simulink model "DUs_Exp"  (R2022b)
settings: Solver=ode4  StartTime=0.0  StopTime=0.3  RelTol=1e-3
model workspace (MAT data in the model file):
  C = 0.0011
  E = 75
  L = 0.001
  R = 10000000
libraries: simulink x30, spsSeriesRLCBranchLib x6, spsCurrentMeasurementLib x4, spsVoltageMeasurementLib x4, spsControlledVoltageSourceLib x2, spsDiodeLib x2, spsMosfetLib x2, spsPWMGeneratorDCDCLib x2, spsStairGeneratorLib x2, spsControlledCurrentSourceLib x1, rllib x1, spspowerguiLib x1
settings Model: Creator=86177  LastModifiedBy=Sweet_J

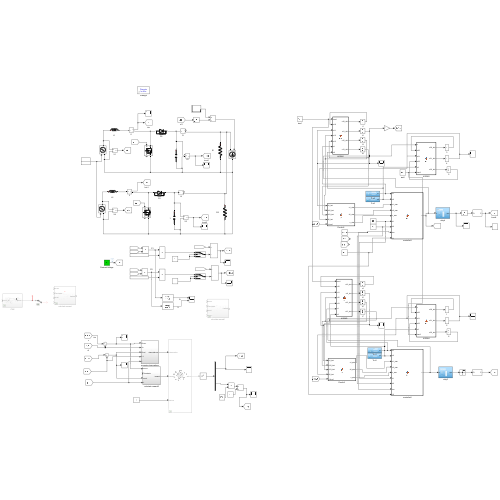
[thumbnail: Simulink's stored preview of the top-level diagram]
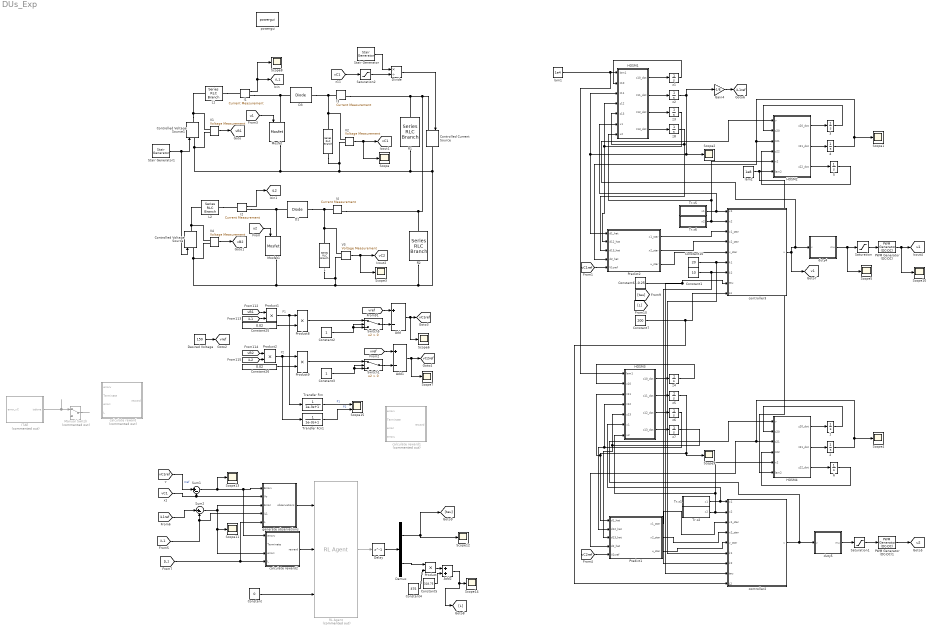
== system DUs_Exp ==
  note: P2
  note: P1
  " " : spsSeriesRLCBranchLib/Series RLC Branch  LConnTagsString=__new0  RConnTagsString=__new0  BranchType=C  Resistance=0.1  Inductance=1e-3  SetiL0=off  InitialCurrent=0  Capacitance=C  Setx0=on  InitialVoltage=150  Measurements=None
  " 1" : spsSeriesRLCBranchLib/Series RLC Branch  LConnTagsString=__new0  RConnTagsString=__new0  BranchType=C  Resistance=0.1  Inductance=1e-3  SetiL0=off  InitialCurrent=0  Capacitance=C  Setx0=off  InitialVoltage=150  Measurements=None
  {1..6} (6 alike) : Integrator  InitialCondition=-5
  Add : Sum  Inputs=+-
  Add1 : Sum  Inputs=+-
  Add2 : Sum
  Constant : Constant  Value=0
  Constant1 : Constant  Value=10
  Constant10 : Constant  Value=20
  Constant2 : Constant
  Constant25 : Constant  Value=0.02
  Constant26 : Constant  Value=0.02
  Constant3 : Constant
  Constant4 : Constant  Value=375
  Constant5 : Constant  Value=318.75
  Constant6 : Constant  Value=-0.25
  Constant7 : Constant  Value=200
  Controlled Current Source : spsControlledCurrentSourceLib/Controlled Current Source  Initialize=on  Source_Type=AC  Amplitude=0  Phase=0  Frequency=0  Measurements=None
  Controlled Voltage Source : spsControlledVoltageSourceLib/Controlled Voltage Source  Initialize=on  Source_Type=DC  Amplitude=0  Phase=0  Frequency=0  Measurements=None
  Controlled Voltage Source1 : spsControlledVoltageSourceLib/Controlled Voltage Source  Initialize=on  Source_Type=DC  Amplitude=0  Phase=0  Frequency=0  Measurements=None
  D1 : spsDiodeLib/Diode  Ron=0.00001  Lon=0  Vf=0  IC=0  UseSnubber=off  Rs=500000  Cs=10e-9  Measurements=off
  D3 : spsDiodeLib/Diode  Ron=0.00001  Lon=0  Vf=0  IC=0  UseSnubber=off  Rs=500000  Cs=10e-9  Measurements=off
  Delay : Delay  DelayLength=1
  Demux : Demux  Outputs=2
  Desired Voltage : Constant  Value=150
  Divide : Product  Inputs=*/
  Gain4 : Gain  Gain=-1/E
  HOSM1 : MATLAB Function  TreatAsAtomicUnit=on
  HOSM2 : MATLAB Function  TreatAsAtomicUnit=on
  HOSM3 : MATLAB Function  TreatAsAtomicUnit=on
  HOSM4 : MATLAB Function  TreatAsAtomicUnit=on
  I{1..4} (4 alike) : spsCurrentMeasurementLib/Current Measurement  PhasorSimulation=off  OutputType=Complex  PSBequivalent=0
  ITAE : Subsystem  Commented=on
  L1 : spsSeriesRLCBranchLib/Series RLC Branch  LConnTagsString=__new0  RConnTagsString=__new0  BranchType=L  Resistance=0.002  Inductance=L  SetiL0=off  InitialCurrent=0  Capacitance=1e-6  Setx0=off  InitialVoltage=0  Measurements=None
  L2 : spsSeriesRLCBranchLib/Series RLC Branch  LConnTagsString=__new0  RConnTagsString=__new0  BranchType=L  Resistance=0.002  Inductance=L  SetiL0=off  InitialCurrent=0  Capacitance=1e-6  Setx0=off  InitialVoltage=0  Measurements=None
  Manual Switch : ManualSwitch  Commented=on
  Mosfet : spsMosfetLib/Mosfet  Ron=0.01  Lon=0  Rd=0.01  Vfd=0  IC=0  Rs=1e5  Cs=inf  Measurements=on
  Mosfet1 : spsMosfetLib/Mosfet  Ron=0.01  Lon=0  Rd=0.01  Vfd=0  IC=0  Rs=1e5  Cs=inf  Measurements=on
  PWM Generator (DC-DC) : spsPWMGeneratorDCDCLib/PWM Generator (DC-DC)  Fsw=20000  Ts=1e-6
  PWM Generator (DC-DC)1 : spsPWMGeneratorDCDCLib/PWM Generator (DC-DC)  Fsw=20000  Ts=1e-6
  Predict1 : MATLAB Function  TreatAsAtomicUnit=on
  Predict2 : MATLAB Function  TreatAsAtomicUnit=on
  Product{,1..2,8..9} (5 alike) : Product
  R1 : spsSeriesRLCBranchLib/Series RLC Branch  LConnTagsString=__new0  RConnTagsString=__new0  BranchType=R  Resistance=R  Inductance=5e-3  SetiL0=off  InitialCurrent=0  Capacitance=1e-6  Setx0=off  InitialVoltage=0  Measurements=None
  R2 : spsSeriesRLCBranchLib/Series RLC Branch  LConnTagsString=__new0  RConnTagsString=__new0  BranchType=R  Resistance=R  Inductance=5e-3  SetiL0=off  InitialCurrent=0  Capacitance=1e-6  Setx0=off  InitialVoltage=0  Measurements=None
  RL Agent : rllib/RL Agent  Commented=on  Agent=agent  ExternalActionAsInput=off  ProvideLastAction=off  ProvideCumRwd=off  TreatAsDirectFeedthrough=on  UseStrictObservationDataTypes=off
  Saturation : Saturate  UpperLimit=0.99  LowerLimit=0.01
  Saturation1 : Saturate  UpperLimit=0.99  LowerLimit=0.01
  Saturation2 : Saturate  UpperLimit=700  LowerLimit=1
  Scope{,1..14} (15 alike) : Scope
  Scope15 : Scope  NumInputPorts=2
  Stair Generator : spsStairGeneratorLib/Stair Generator  t=[0, 0.11, 0.23]  e=[800,100,400]  Ts=0
  Stair Generator1 : spsStairGeneratorLib/Stair Generator  t=[0,0.2,0.25]  e=[75,75,75]  Ts=0
  Sum1 : Sum  Inputs=|+-
  Sum2 : Sum  Inputs=|+-
  Switch1 : Switch  Criteria=u2 > Threshold  SaturateOnIntegerOverflow=off  InputSameDT=off
  Switch5 : Switch  Criteria=u2 > Threshold  SaturateOnIntegerOverflow=off  InputSameDT=off
  Tr.x1 : Subsystem
  Tr.x2 : Subsystem
  Tr.x5 : Subsystem
  Tr.x6 : Subsystem
  Transfer Fcn : TransferFcn  Denominator=[1e-3 1]
  Transfer Fcn1 : TransferFcn  Denominator=[1e-3 1]
  V{1..4} (4 alike) : spsVoltageMeasurementLib/Voltage Measurement  PhasorSimulation=off  OutputType=Complex  PSBequivalent=0
  calculate reward : Subsystem  Commented=on
  calculate reward1 : Subsystem  Commented=on
  calculate reward2 : Subsystem
  controller2 : MATLAB Function  TreatAsAtomicUnit=on
  controller3 : MATLAB Function  TreatAsAtomicUnit=on
  duty4 : Subsystem
  duty5 : Subsystem
  generate observations : Subsystem
  lam1 : Constant  Value=1e4
  lam2 : Constant  Value=1e8
  powergui : spspowerguiLib/powergui  Priority=1  SimulationMode=Discrete  SampleTime=1e-6  frequency=60  Iterations=50  frequencyindice=0  Pbase=100e6  ErrMax=1e-4  UnitsV=kV  UnitsW=MW  buscounter=0  FunctionMessages=off  echomessages=off  EnableUseOfTLC=off  CurrentSourceSwitches=off  DisableSnubberDevices=off  DisableRonSwitches=off  DisableVfSwitches=off  DisplayEquations=off  AutomaticDiscreteSolvers=off  SolverType=Tustin/Backward Euler (TBE)  Interpol=off  ExternalGateDelay=off  methode=off  Ts=100  x0status=blocks  SPID=on  SwTol=0  HookPort=off  NonlinearTolerance=1e-4  nMaxIteration=100  ContinueOnMaxIteration=off  RestoreLinks=warning  ResistiveCurrentMeasurement=off  Frange=[0:2:500]  Ylog=off  Xlog=on  ShowGrid=off  save=off  variable=ZData  structure=0  ZoomFFT=off  StartTime=0.0  cycles=1  DisplayStyle=1  fundamental=60  FreqAxis=off  MaxFrequency=1000  frequencyindicesteady=1  RmsSteady=1  display=off
  z1 : Integrator  InitialCondition=-1
  z2 : Integrator  InitialCondition=-200
  z{3,6..8} (4 alike) : Integrator
  z4 : Integrator  InitialCondition=-1
  z5 : Integrator  InitialCondition=-200
  tag scope: iL1=global, iL1ref=global, iL2=global, u1=global, u2=global, v1=global, vB1=global, vB2=global, vC1=global, vC1ref=global, vC2=global, vC2ref=global, vref=global
  wires:
  Manual Switch/1 -> ?
  Add2/1 -> [L], Scope14/1
  RL Agent/1 -> Delay/1
  Sum1/1 -> Scope13/1, calculate reward2/1(errorv), generate observations/1(Errorv)
  ITAE/1(isdone) -> Manual Switch/1
  4/1 -> Scope1/1, Predict2/4(d2_hat), HOSM2/3(z21)
  I1/1 -> [iL1], Scope8/1
  V2/1 -> [vC1], Scope/1
  Stair Generator1/1 -> Controlled Voltage Source/1, Controlled Voltage Source1/1
  Divide/1 -> Controlled Current Source/1
  Gain4/1 -> [iL1ref]
  [vC1ref] -> Sum1/1  "Vref"
  calculate reward2/1(reward) -> RL Agent/2
  Tr.x1/1(x1) -> HOSM3/6(x1), controller2/1(x1)
  generate observations/1(observations) -> RL Agent/1
  [vC1] -> Sum1/2, generate observations/2(Vo)
  Constant3/1 -> Switch1/3, Switch1/2
  [iL1] -> generate observations/4(iL1), Sum2/2
  Sum2/1 -> calculate reward2/3(errori), Scope11/1, generate observations/3(Errori)
  [vC1] -> Saturation2/1
  duty5/1(mu) -> Saturation1/1
  Saturation/1 -> PWM Generator (DC-DC)/1
  Add1/1 -> [vC2ref], Scope7/1
  Predict2/3(u_star) -> controller3/5(v_star)
  HOSM3/1(z10_dot) -> z4/1
  HOSM2/2(z21_dot) -> 4/1
  Constant10/1 -> controller2/6(k1), controller3/6(k1)
  controller3/1(v) -> duty4/1(v), HOSM2/1(v), [v1]
  Saturation1/1 -> PWM Generator (DC-DC)1/1
  Add/1 -> [vC1ref], Scope6/1
  Saturation2/1 -> Divide/2
  duty4/1(mu) -> Scope5/1, Saturation/1
  Constant25/1 -> Product8/2
  Tr.x6/1(x2) -> HOSM1/7(x2), HOSM2/5(x2), controller3/2(x2)
  Predict1/3(u_star) -> controller2/5(v_star)
  z4/1 -> HOSM3/2(z10)
  [vC2ref] -> Predict1/5(V2cref)
  V1/1 -> [vB1]
  HOSM1/4(z13_dot) -> z8/1
  I2/1 -> [iL2]
  Predict2/2(x2_star) -> controller3/4(x2_star)
  Desired Voltage/1 -> [vref]
  3/1 -> HOSM2/2(z20)
  z3/1 -> Predict2/2(d12_hat), HOSM1/4(z12)
  HOSM2/3(z22_dot) -> 5/1
  HOSM2/1(z20_dot) -> 3/1
  5/1 -> HOSM2/4(z22)
  z1/1 -> HOSM1/2(z10)
  HOSM1/2(z11_dot) -> z2/1
  [iL1ref] -> Sum2/1
  PWM Generator (DC-DC)1/1 -> [u2]
  z8/1 -> Predict2/3(d13_hat), HOSM1/5(z13)
  Constant26/1 -> Product9/2
  Predict2/1(x1_star) -> controller3/3(x1_star)
  [vB1] -> Product1/1
  [vB2] -> Product2/1
  Constant2/1 -> Switch5/2, Switch5/3
  HOSM4/3(z22_dot) -> 6/1
  HOSM1/1(z10_dot) -> z1/1
  [iL1] -> Product1/2
  PWM Generator (DC-DC)/1 -> [u1], Scope10/1
  Switch5/1 -> Add/2
  [vref] -> Add1/1
  Product2/1 -> Product9/1, Transfer Fcn1/1
  Stair Generator/1 -> Divide/1
  6/1 -> HOSM4/4(z22)
  lam1/1 -> HOSM3/1(lam1), HOSM1/1(lam1)
  1/1 -> HOSM4/2(z20)
  z6/1 -> HOSM3/4(z12), Predict1/2(d12_hat)
  HOSM3/3(z12_dot) -> z6/1
  V4/1 -> [vB2]
  HOSM1/3(z12_dot) -> z3/1
  Switch1/1 -> Add1/2
  Product9/1 -> Switch1/1
  [iL2] -> Product2/2
  Product8/1 -> Switch5/1
  Predict1/2(x2_star) -> controller2/4(x2_star)
  Constant1/1 -> controller2/7(k2), controller3/7(k2)
  HOSM3/2(z11_dot) -> z5/1
  HOSM4/2(z21_dot) -> 2/1
  Tr.x5/1(x1) -> HOSM1/6(x1), controller3/1(x1)
  2/1 -> HOSM4/3(z21), Predict1/4(d2_hat), Scope4/1
  z7/1 -> HOSM3/5(z13), Predict1/3(d13_hat)
  V3/1 -> [vC2], Scope3/1
  controller2/1(v) -> HOSM4/1(v), duty5/1(v)
  Product1/1 -> Product8/1, Transfer Fcn/1
  Tr.x2/1(x2) -> controller2/2(x2), HOSM4/5(x2), HOSM3/7(x2)
  [vref] -> Add/1
  HOSM4/1(z20_dot) -> 1/1
  Predict1/1(x1_star) -> controller2/3(x1_star)
  [vC1ref] -> Predict2/5(V1cref)
  z2/1 -> Scope2/1, HOSM1/3(z11), Predict2/1(d1_hat), Gain4/1
  HOSM3/4(z13_dot) -> z7/1
  z5/1 -> Scope9/1, Predict1/1(d1_hat), HOSM3/3(z11)
  [u1] -> Mosfet/1
  lam2/1 -> HOSM4/6(lam2), HOSM2/6(lam2)
  Demux/1 -> Scope12/1, [tau]
  [u2] -> Mosfet1/1
  Delay/1 -> Demux/1
  Demux/2 -> Product/1
  Constant4/1 -> Product/2
  Product/1 -> Add2/1
  Constant5/1 -> Add2/2
  Constant6/1 -> controller3/8(tau), controller2/8(tau)
  Constant/1 -> RL Agent/3
  Transfer Fcn/1 -> Scope15/1  "P1"
  Transfer Fcn1/1 -> Scope15/2  "P2"
  [L] -> calculate reward2/4(L), generate observations/5(L)
  Constant7/1 -> controller2/9(L2), controller3/9(L1)
  connections:
  Controlled Voltage Source1/RConn1 -- V1/LConn1 -- L1/LConn1
  L2/LConn1 -- Controlled Voltage Source/RConn1 -- V4/LConn1
  V2/LConn1 -- D3/RConn1 -- I3/LConn1 -- " "/LConn1
  " 1"/LConn1 -- V3/LConn1 -- D1/RConn1 -- I4/LConn1
  I1/RConn1 -- D3/LConn1 -- Mosfet/LConn1
  Mosfet1/LConn1 -- I2/RConn1 -- D1/LConn1
  L2/RConn1 -- I2/LConn1
  L1/RConn1 -- I1/LConn1
  I3/RConn1 -- I4/RConn1 -- R2/LConn1 -- Controlled Current Source/LConn1 -- R1/LConn1
  R2/RConn1 -- R1/RConn1 -- Controlled Voltage Source1/LConn1 -- V1/LConn2 -- Mosfet/RConn1 -- " "/RConn1 -- V2/LConn2 -- Controlled Current Source/RConn1 -- V3/LConn2 -- " 1"/RConn1 -- Controlled Voltage Source/LConn1 -- V4/LConn2 -- Mosfet1/RConn1

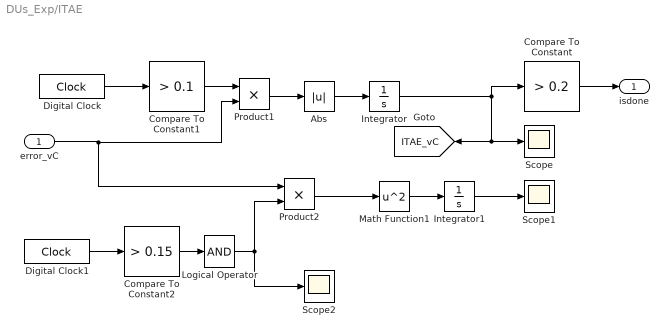
== system DUs_Exp/ITAE ==
  error_vC : Inport
  Abs : Abs  ZeroCross=off  SaturateOnIntegerOverflow=off
  Compare To Constant : simulink/Logic and Bit Operations/Compare To Constant  relop=>  const=0.2  OutDataTypeStr=boolean  ZeroCross=off
  Compare To Constant1 : simulink/Logic and Bit Operations/Compare To Constant  relop=>  const=0.1  OutDataTypeStr=boolean  ZeroCross=off
  Compare To Constant2 : simulink/Logic and Bit Operations/Compare To Constant  relop=>  const=0.15  OutDataTypeStr=boolean  ZeroCross=off
  Digital Clock : DigitalClock  SampleTime=1e-6
  Digital Clock1 : DigitalClock  SampleTime=1e-6
  Integrator : Integrator
  Integrator1 : Integrator
  Logical Operator : Logic  Inputs=1  AllPortsSameDT=off  OutDataTypeStr=boolean
  Math Function1 : Math  Operator=square
  Product1 : Product
  Product2 : Product
  Scope : Scope
  Scope1 : Scope
  Scope2 : Scope
  isdone : Outport
  tag scope: ITAE_vC=global
  wires:
  Abs/1 -> Integrator/1
  Digital Clock/1 -> Compare To Constant1/1
  Product1/1 -> Abs/1
  Compare To Constant/1 -> isdone/1
  Math Function1/1 -> Integrator1/1
  Integrator/1 -> Scope/1, [ITAE_vC], Compare To Constant/1
  Compare To Constant1/1 -> Product1/1
  Integrator1/1 -> Scope1/1
  Compare To Constant2/1 -> Logical Operator/1
  Digital Clock1/1 -> Compare To Constant2/1
  Logical Operator/1 -> Scope2/1, Product2/2
  error_vC/1 -> Product2/1, Product1/2
  Product2/1 -> Math Function1/1

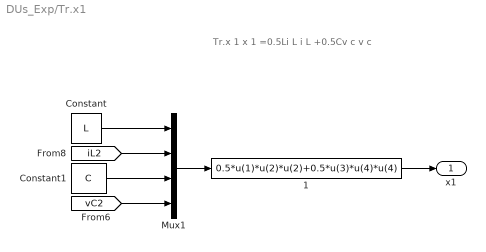
== system DUs_Exp/Tr.x1 ==
  note: Tr.x 1
      | x 1 =0.5Li L i L +0.5Cv c v c
  1 : Fcn  Expr=0.5*u(1)*u(2)*u(2)+0.5*u(3)*u(4)*u(4)
  Constant : Constant  Value=L
  Constant1 : Constant  Value=C
  Mux1 : Mux
  x1 : Outport  VectorParamsAs1DForOutWhenUnconnected=off
  wires:
  1/1 -> x1/1
  Mux1/1 -> 1/1
  Constant/1 -> Mux1/1
  [iL2] -> Mux1/2
  Constant1/1 -> Mux1/3
  [vC2] -> Mux1/4

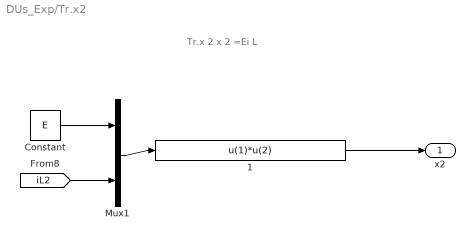
== system DUs_Exp/Tr.x2 ==
  note: Tr.x 2
      | x 2 =Ei L
  1 : Fcn  Expr=u(1)*u(2)
  Constant : Constant  Value=E
  Mux1 : Mux  Inputs=2
  x2 : Outport  VectorParamsAs1DForOutWhenUnconnected=off
  wires:
  [iL2] -> Mux1/2
  Mux1/1 -> 1/1
  1/1 -> x2/1
  Constant/1 -> Mux1/1

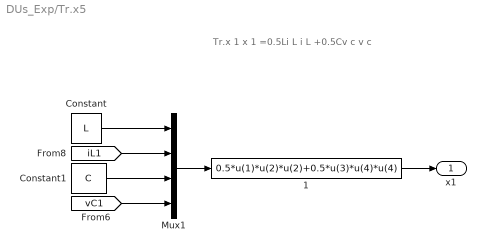
== system DUs_Exp/Tr.x5 ==
  note: Tr.x 1
      | x 1 =0.5Li L i L +0.5Cv c v c
  1 : Fcn  Expr=0.5*u(1)*u(2)*u(2)+0.5*u(3)*u(4)*u(4)
  Constant : Constant  Value=L
  Constant1 : Constant  Value=C
  Mux1 : Mux
  x1 : Outport  VectorParamsAs1DForOutWhenUnconnected=off
  wires:
  1/1 -> x1/1
  Mux1/1 -> 1/1
  Constant/1 -> Mux1/1
  [iL1] -> Mux1/2
  Constant1/1 -> Mux1/3
  [vC1] -> Mux1/4

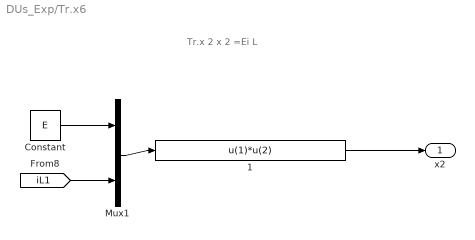
== system DUs_Exp/Tr.x6 ==
  note: Tr.x 2
      | x 2 =Ei L
  1 : Fcn  Expr=u(1)*u(2)
  Constant : Constant  Value=E
  Mux1 : Mux  Inputs=2
  x2 : Outport  VectorParamsAs1DForOutWhenUnconnected=off
  wires:
  [iL1] -> Mux1/2
  Mux1/1 -> 1/1
  1/1 -> x2/1
  Constant/1 -> Mux1/1

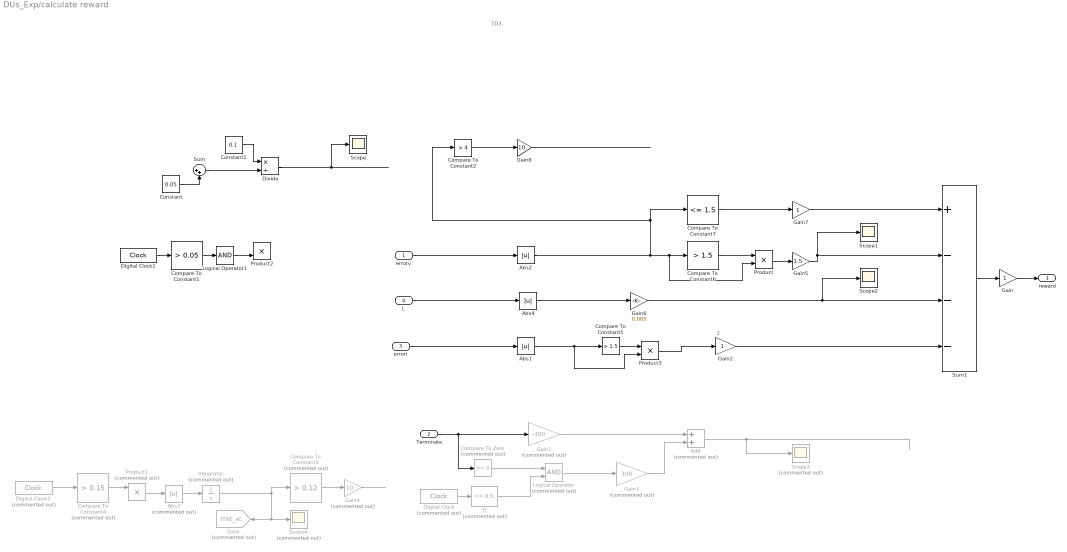
== system DUs_Exp/calculate reward ==
  note: 2
  note: TD3
  errorv : Inport
  Terminate : Inport  Port=2
  errori : Inport  Port=3
  L : Inport  Port=4
  Abs1 : Abs  ZeroCross=off  SaturateOnIntegerOverflow=off
  Abs2 : Abs  ZeroCross=off  SaturateOnIntegerOverflow=off
  Abs3 : Abs  Commented=on  ZeroCross=off  SaturateOnIntegerOverflow=off
  Abs4 : Abs  ZeroCross=off  SaturateOnIntegerOverflow=off
  Add : Sum  Commented=on
  Compare To Constant1 : simulink/Logic and Bit Operations/Compare To Constant  relop=>  const=0.05  OutDataTypeStr=boolean  ZeroCross=off
  Compare To Constant2 : simulink/Logic and Bit Operations/Compare To Constant  relop=>  const=4  OutDataTypeStr=boolean
  Compare To Constant3 : simulink/Logic and Bit Operations/Compare To Constant  Commented=on  relop=>  const=0.12  OutDataTypeStr=boolean  ZeroCross=off
  Compare To Constant4 : simulink/Logic and Bit Operations/Compare To Constant  Commented=on  relop=>  const=0.15  OutDataTypeStr=boolean  ZeroCross=off
  Compare To Constant5 : simulink/Logic and Bit Operations/Compare To Constant  relop=>  const=1.5  OutDataTypeStr=boolean
  Compare To Constant6 : simulink/Logic and Bit Operations/Compare To Constant  relop=>  const=1.5  OutDataTypeStr=boolean  ZeroCross=off
  Compare To Constant7 : simulink/Logic and Bit Operations/Compare To Constant  relop=<=  const=1.5  OutDataTypeStr=boolean  ZeroCross=off
  Compare To Zero : simulink/Logic and Bit Operations/Compare To Zero  Commented=on  relop===  OutDataTypeStr=boolean
  Constant : Constant  Value=0.05
  Constant1 : Constant  Value=0.1
  Digital Clock : DigitalClock  Commented=on  SampleTime=1e-6
  Digital Clock1 : DigitalClock  SampleTime=1e-6
  Digital Clock2 : DigitalClock  Commented=on  SampleTime=1e-6
  Divide : Product  Inputs=*/
  Gain : Gain
  Gain1 : Gain  Commented=on  Gain=-100
  Gain2 : Gain
  Gain3 : Gain  Commented=on  Gain=100
  Gain4 : Gain  Commented=on  Gain=10
  Gain5 : Gain  Gain=1.5
  Gain6 : Gain  Gain=0.005
  Gain7 : Gain
  Gain8 : Gain  Gain=10
  Goto : Goto  Commented=on  GotoTag=ITAE_vC  TagVisibility=global
  Integrator : Integrator  Commented=on
  Logical Operator : Logic  Commented=on  AllPortsSameDT=off  OutDataTypeStr=boolean
  Logical Operator1 : Logic  Inputs=1  AllPortsSameDT=off  OutDataTypeStr=boolean
  Product : Product
  Product1 : Product  Commented=on
  Product2 : Product
  Product3 : Product
  Scope : Scope
  Scope1 : Scope
  Scope2 : Scope
  Scope3 : Scope  Commented=on
  Scope4 : Scope  Commented=on
  Sum : Sum  Inputs=|++
  Sum1 : Sum  Inputs=+---  OutDataTypeStr=double
  Tf : simulink/Logic and Bit Operations/Compare To Constant  Commented=on  relop===  const=0.5  OutDataTypeStr=boolean  ZeroCross=off
  reward : Outport  VectorParamsAs1DForOutWhenUnconnected=off
  wires:
  Sum/1 -> Divide/2
  Constant/1 -> Sum/2
  Constant1/1 -> Divide/1
  Gain5/1 -> Sum1/2, Scope1/1
  Sum1/1 -> Gain/1
  Divide/1 -> Scope/1
  Gain/1 -> reward/1
  Gain1/1 -> Add/1
  Gain3/1 -> Add/2
  Compare To Zero/1 -> Logical Operator/1
  Digital Clock/1 -> Tf/1
  Terminate/1 -> Compare To Zero/1, Gain1/1
  Tf/1 -> Logical Operator/2
  Logical Operator/1 -> Gain3/1
  errori/1 -> Abs1/1
  Compare To Constant2/1 -> Gain8/1
  Gain2/1 -> Sum1/4
  Add/1 -> Scope3/1
  Logical Operator1/1 -> Product2/2
  Compare To Constant1/1 -> Logical Operator1/1
  Digital Clock1/1 -> Compare To Constant1/1
  errorv/1 -> Abs2/1
  Abs2/1 -> Compare To Constant2/1, Compare To Constant7/1, Product/2, Compare To Constant6/1
  Integrator/1 -> Goto/1, Scope4/1, Compare To Constant3/1
  Abs3/1 -> Integrator/1
  Digital Clock2/1 -> Compare To Constant4/1
  Compare To Constant3/1 -> Gain4/1
  Product1/1 -> Abs3/1
  Compare To Constant4/1 -> Product1/1
  Gain4/1 -> ?
  Gain8/1 -> ?
  Product3/1 -> Gain2/1
  L/1 -> Abs4/1
  Gain6/1 -> Sum1/3, Scope2/1
  Abs4/1 -> Gain6/1
  Abs1/1 -> Product3/2, Compare To Constant5/1
  Product/1 -> Gain5/1
  Compare To Constant7/1 -> Gain7/1
  Gain7/1 -> Sum1/1
  Compare To Constant6/1 -> Product/1
  Compare To Constant5/1 -> Product3/1

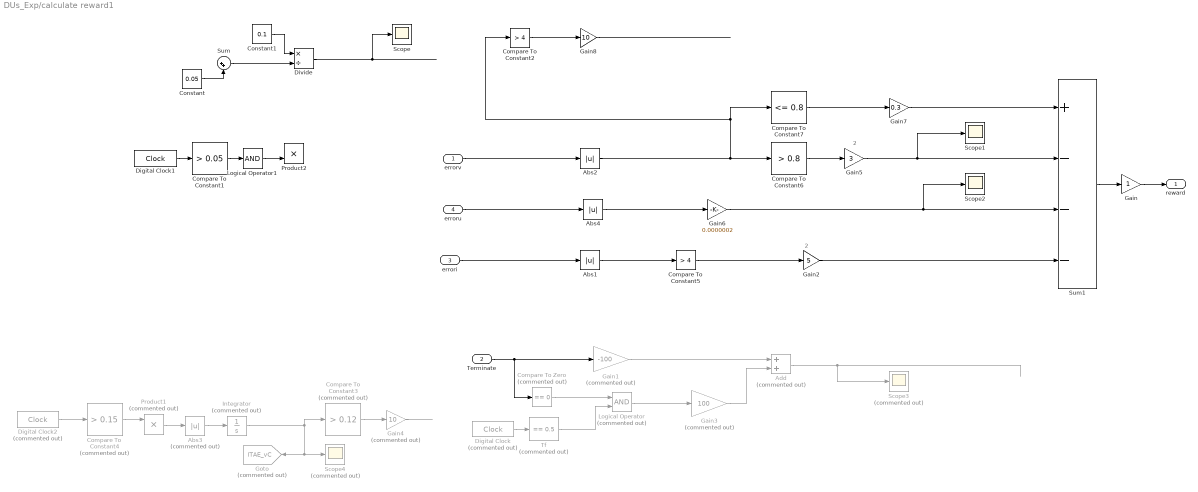
== system DUs_Exp/calculate reward1 ==
  note: 2
  note: 2
  errorv : Inport
  Terminate : Inport  Port=2
  errori : Inport  Port=3
  erroru : Inport  Port=4
  Abs1 : Abs  ZeroCross=off  SaturateOnIntegerOverflow=off
  Abs2 : Abs  ZeroCross=off  SaturateOnIntegerOverflow=off
  Abs3 : Abs  Commented=on  ZeroCross=off  SaturateOnIntegerOverflow=off
  Abs4 : Abs  ZeroCross=off  SaturateOnIntegerOverflow=off
  Add : Sum  Commented=on
  Compare To Constant1 : simulink/Logic and Bit Operations/Compare To Constant  relop=>  const=0.05  OutDataTypeStr=boolean  ZeroCross=off
  Compare To Constant2 : simulink/Logic and Bit Operations/Compare To Constant  relop=>  const=4  OutDataTypeStr=boolean
  Compare To Constant3 : simulink/Logic and Bit Operations/Compare To Constant  Commented=on  relop=>  const=0.12  OutDataTypeStr=boolean  ZeroCross=off
  Compare To Constant4 : simulink/Logic and Bit Operations/Compare To Constant  Commented=on  relop=>  const=0.15  OutDataTypeStr=boolean  ZeroCross=off
  Compare To Constant5 : simulink/Logic and Bit Operations/Compare To Constant  relop=>  const=4  OutDataTypeStr=boolean
  Compare To Constant6 : simulink/Logic and Bit Operations/Compare To Constant  relop=>  const=0.8  OutDataTypeStr=boolean  ZeroCross=off
  Compare To Constant7 : simulink/Logic and Bit Operations/Compare To Constant  relop=<=  const=0.8  OutDataTypeStr=boolean  ZeroCross=off
  Compare To Zero : simulink/Logic and Bit Operations/Compare To Zero  Commented=on  relop===  OutDataTypeStr=boolean
  Constant : Constant  Value=0.05
  Constant1 : Constant  Value=0.1
  Digital Clock : DigitalClock  Commented=on  SampleTime=1e-6
  Digital Clock1 : DigitalClock  SampleTime=1e-6
  Digital Clock2 : DigitalClock  Commented=on  SampleTime=1e-6
  Divide : Product  Inputs=*/
  Gain : Gain
  Gain1 : Gain  Commented=on  Gain=-100
  Gain2 : Gain  Gain=5
  Gain3 : Gain  Commented=on  Gain=100
  Gain4 : Gain  Commented=on  Gain=10
  Gain5 : Gain  Gain=3
  Gain6 : Gain  Gain=0.0000002
  Gain7 : Gain  Gain=0.3
  Gain8 : Gain  Gain=10
  Goto : Goto  Commented=on  GotoTag=ITAE_vC  TagVisibility=global
  Integrator : Integrator  Commented=on
  Logical Operator : Logic  Commented=on  AllPortsSameDT=off  OutDataTypeStr=boolean
  Logical Operator1 : Logic  Inputs=1  AllPortsSameDT=off  OutDataTypeStr=boolean
  Product1 : Product  Commented=on
  Product2 : Product
  Scope : Scope
  Scope1 : Scope
  Scope2 : Scope
  Scope3 : Scope  Commented=on
  Scope4 : Scope  Commented=on
  Sum : Sum  Inputs=|++
  Sum1 : Sum  Inputs=+---  OutDataTypeStr=double
  Tf : simulink/Logic and Bit Operations/Compare To Constant  Commented=on  relop===  const=0.5  OutDataTypeStr=boolean  ZeroCross=off
  reward : Outport  VectorParamsAs1DForOutWhenUnconnected=off
  wires:
  Gain7/1 -> Sum1/1
  Compare To Constant7/1 -> Gain7/1
  Compare To Constant6/1 -> Gain5/1
  Abs1/1 -> Compare To Constant5/1
  Abs4/1 -> Gain6/1
  Gain6/1 -> Scope2/1, Sum1/3
  erroru/1 -> Abs4/1
  Compare To Constant5/1 -> Gain2/1
  Gain8/1 -> ?
  Gain4/1 -> ?
  Compare To Constant4/1 -> Product1/1
  Product1/1 -> Abs3/1
  Compare To Constant3/1 -> Gain4/1
  Digital Clock2/1 -> Compare To Constant4/1
  Abs3/1 -> Integrator/1
  Integrator/1 -> Compare To Constant3/1, Scope4/1, Goto/1
  Abs2/1 -> Compare To Constant6/1, Compare To Constant7/1, Compare To Constant2/1
  errorv/1 -> Abs2/1
  Digital Clock1/1 -> Compare To Constant1/1
  Compare To Constant1/1 -> Logical Operator1/1
  Logical Operator1/1 -> Product2/2
  Add/1 -> Scope3/1
  Gain2/1 -> Sum1/4
  Compare To Constant2/1 -> Gain8/1
  errori/1 -> Abs1/1
  Logical Operator/1 -> Gain3/1
  Tf/1 -> Logical Operator/2
  Terminate/1 -> Gain1/1, Compare To Zero/1
  Digital Clock/1 -> Tf/1
  Compare To Zero/1 -> Logical Operator/1
  Gain3/1 -> Add/2
  Gain1/1 -> Add/1
  Gain/1 -> reward/1
  Divide/1 -> Scope/1
  Sum1/1 -> Gain/1
  Gain5/1 -> Scope1/1, Sum1/2
  Constant1/1 -> Divide/1
  Constant/1 -> Sum/2
  Sum/1 -> Divide/2

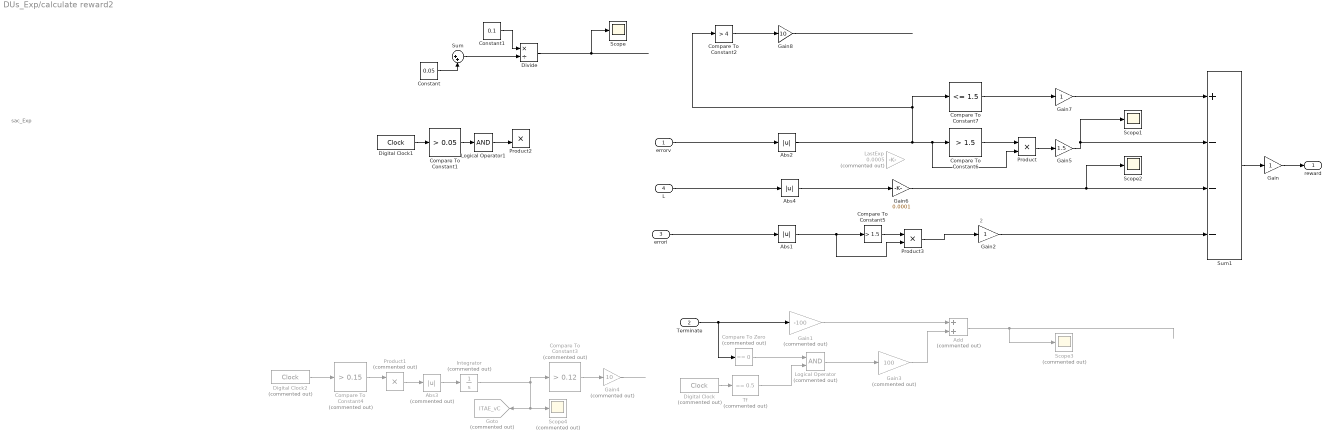
== system DUs_Exp/calculate reward2 ==
  note: sac_Exp
  note: 2
  errorv : Inport
  Terminate : Inport  Port=2
  errori : Inport  Port=3
  L : Inport  Port=4
  Abs1 : Abs  ZeroCross=off  SaturateOnIntegerOverflow=off
  Abs2 : Abs  ZeroCross=off  SaturateOnIntegerOverflow=off
  Abs3 : Abs  Commented=on  ZeroCross=off  SaturateOnIntegerOverflow=off
  Abs4 : Abs  ZeroCross=off  SaturateOnIntegerOverflow=off
  Add : Sum  Commented=on
  Compare To Constant1 : simulink/Logic and Bit Operations/Compare To Constant  relop=>  const=0.05  OutDataTypeStr=boolean  ZeroCross=off
  Compare To Constant2 : simulink/Logic and Bit Operations/Compare To Constant  relop=>  const=4  OutDataTypeStr=boolean
  Compare To Constant3 : simulink/Logic and Bit Operations/Compare To Constant  Commented=on  relop=>  const=0.12  OutDataTypeStr=boolean  ZeroCross=off
  Compare To Constant4 : simulink/Logic and Bit Operations/Compare To Constant  Commented=on  relop=>  const=0.15  OutDataTypeStr=boolean  ZeroCross=off
  Compare To Constant5 : simulink/Logic and Bit Operations/Compare To Constant  relop=>  const=1.5  OutDataTypeStr=boolean
  Compare To Constant6 : simulink/Logic and Bit Operations/Compare To Constant  relop=>  const=1.5  OutDataTypeStr=boolean  ZeroCross=off
  Compare To Constant7 : simulink/Logic and Bit Operations/Compare To Constant  relop=<=  const=1.5  OutDataTypeStr=boolean  ZeroCross=off
  Compare To Zero : simulink/Logic and Bit Operations/Compare To Zero  Commented=on  relop===  OutDataTypeStr=boolean
  Constant : Constant  Value=0.05
  Constant1 : Constant  Value=0.1
  Digital Clock : DigitalClock  Commented=on  SampleTime=1e-6
  Digital Clock1 : DigitalClock  SampleTime=1e-6
  Digital Clock2 : DigitalClock  Commented=on  SampleTime=1e-6
  Divide : Product  Inputs=*/
  Gain : Gain
  Gain1 : Gain  Commented=on  Gain=-100
  Gain2 : Gain
  Gain3 : Gain  Commented=on  Gain=100
  Gain4 : Gain  Commented=on  Gain=10
  Gain5 : Gain  Gain=1.5
  Gain6 : Gain  Gain=0.0001
  Gain7 : Gain
  Gain8 : Gain  Gain=10
  Goto : Goto  Commented=on  GotoTag=ITAE_vC  TagVisibility=global
  Integrator : Integrator  Commented=on
  LastExp : Gain  Commented=on  Gain=0.0005
  Logical Operator : Logic  Commented=on  AllPortsSameDT=off  OutDataTypeStr=boolean
  Logical Operator1 : Logic  Inputs=1  AllPortsSameDT=off  OutDataTypeStr=boolean
  Product : Product
  Product1 : Product  Commented=on
  Product2 : Product
  Product3 : Product
  Scope : Scope
  Scope1 : Scope
  Scope2 : Scope
  Scope3 : Scope  Commented=on
  Scope4 : Scope  Commented=on
  Sum : Sum  Inputs=|++
  Sum1 : Sum  Inputs=+---  OutDataTypeStr=double
  Tf : simulink/Logic and Bit Operations/Compare To Constant  Commented=on  relop===  const=0.5  OutDataTypeStr=boolean  ZeroCross=off
  reward : Outport  VectorParamsAs1DForOutWhenUnconnected=off
  wires:
  Compare To Constant5/1 -> Product3/1
  Compare To Constant6/1 -> Product/1
  Gain7/1 -> Sum1/1
  Compare To Constant7/1 -> Gain7/1
  Product/1 -> Gain5/1
  Abs1/1 -> Compare To Constant5/1, Product3/2
  Abs4/1 -> Gain6/1
  Gain6/1 -> Scope2/1, Sum1/3
  L/1 -> Abs4/1
  Product3/1 -> Gain2/1
  Gain8/1 -> ?
  Gain4/1 -> ?
  Compare To Constant4/1 -> Product1/1
  Product1/1 -> Abs3/1
  Compare To Constant3/1 -> Gain4/1
  Digital Clock2/1 -> Compare To Constant4/1
  Abs3/1 -> Integrator/1
  Integrator/1 -> Compare To Constant3/1, Scope4/1, Goto/1
  Abs2/1 -> Compare To Constant6/1, Product/2, Compare To Constant7/1, Compare To Constant2/1
  errorv/1 -> Abs2/1
  Digital Clock1/1 -> Compare To Constant1/1
  Compare To Constant1/1 -> Logical Operator1/1
  Logical Operator1/1 -> Product2/2
  Add/1 -> Scope3/1
  Gain2/1 -> Sum1/4
  Compare To Constant2/1 -> Gain8/1
  errori/1 -> Abs1/1
  Logical Operator/1 -> Gain3/1
  Tf/1 -> Logical Operator/2
  Terminate/1 -> Gain1/1, Compare To Zero/1
  Digital Clock/1 -> Tf/1
  Compare To Zero/1 -> Logical Operator/1
  Gain3/1 -> Add/2
  Gain1/1 -> Add/1
  Gain/1 -> reward/1
  Divide/1 -> Scope/1
  Sum1/1 -> Gain/1
  Gain5/1 -> Scope1/1, Sum1/2
  Constant1/1 -> Divide/1
  Constant/1 -> Sum/2
  Sum/1 -> Divide/2

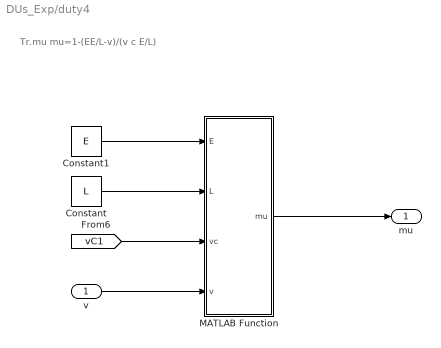
== system DUs_Exp/duty4 ==
  note: Tr.mu
      | mu=1-(EE/L-v)/(v c E/L)
  v : Inport
  Constant : Constant  Value=L
  Constant1 : Constant  Value=E
  MATLAB Function : MATLAB Function  TreatAsAtomicUnit=on
  mu : Outport  VectorParamsAs1DForOutWhenUnconnected=off
  wires:
  MATLAB Function/1(mu) -> mu/1
  v/1 -> MATLAB Function/4(v)
  [vC1] -> MATLAB Function/3(vc)
  Constant/1 -> MATLAB Function/2(L)
  Constant1/1 -> MATLAB Function/1(E)

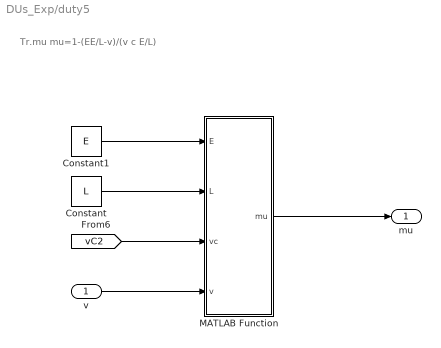
== system DUs_Exp/duty5 ==
  note: Tr.mu
      | mu=1-(EE/L-v)/(v c E/L)
  v : Inport
  Constant : Constant  Value=L
  Constant1 : Constant  Value=E
  MATLAB Function : MATLAB Function  TreatAsAtomicUnit=on
  mu : Outport  VectorParamsAs1DForOutWhenUnconnected=off
  wires:
  Constant1/1 -> MATLAB Function/1(E)
  Constant/1 -> MATLAB Function/2(L)
  [vC2] -> MATLAB Function/3(vc)
  v/1 -> MATLAB Function/4(v)
  MATLAB Function/1(mu) -> mu/1

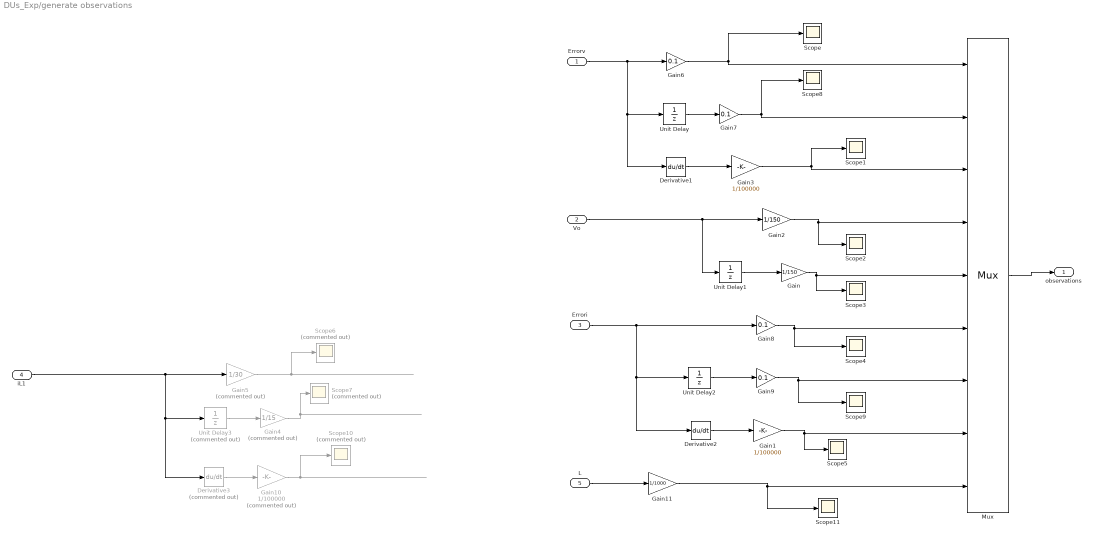
== system DUs_Exp/generate observations ==
  Errorv : Inport
  Vo : Inport  Port=2
  Errori : Inport  Port=3
  iL1 : Inport  Port=4
  L : Inport  Port=5
  Derivative1 : Derivative
  Derivative2 : Derivative
  Derivative3 : Derivative  Commented=on
  Gain : Gain  Gain=1/150
  Gain1 : Gain  Gain=1/100000
  Gain10 : Gain  Commented=on  Gain=1/100000
  Gain11 : Gain  Gain=1/1000
  Gain2 : Gain  Gain=1/150
  Gain3 : Gain  Gain=1/100000
  Gain4 : Gain  Commented=on  Gain=1/15
  Gain5 : Gain  Commented=on  Gain=1/30
  Gain{6..9} (4 alike) : Gain  Gain=0.1
  Mux : Mux  Inputs=9
  Scope{,1..5,8..9,11} (9 alike) : Scope
  Scope10 : Scope  Commented=on
  Scope6 : Scope  Commented=on
  Scope7 : Scope  Commented=on
  Unit Delay : UnitDelay  SampleTime=-1  HasFrameUpgradeWarning=on
  Unit Delay1 : UnitDelay  SampleTime=-1  HasFrameUpgradeWarning=on
  Unit Delay2 : UnitDelay  SampleTime=-1  HasFrameUpgradeWarning=on
  Unit Delay3 : UnitDelay  Commented=on  SampleTime=-1  HasFrameUpgradeWarning=on
  observations : Outport  VectorParamsAs1DForOutWhenUnconnected=off
  wires:
  Mux/1 -> observations/1
  Errorv/1 -> Derivative1/1, Unit Delay/1, Gain6/1
  Vo/1 -> Unit Delay1/1, Gain2/1
  Unit Delay1/1 -> Gain/1
  Gain/1 -> Scope3/1, Mux/5
  Derivative1/1 -> Gain3/1
  Gain3/1 -> Scope1/1, Mux/3
  Gain2/1 -> Scope2/1, Mux/4
  Gain1/1 -> Scope5/1, Mux/8
  Derivative2/1 -> Gain1/1
  Errori/1 -> Derivative2/1, Unit Delay2/1, Gain8/1
  Gain5/1 -> Scope6/1
  Gain4/1 -> Scope7/1
  Unit Delay3/1 -> Gain4/1
  Gain6/1 -> Scope/1, Mux/1
  Unit Delay/1 -> Gain7/1
  Gain7/1 -> Scope8/1, Mux/2
  Gain8/1 -> Scope4/1, Mux/6
  Unit Delay2/1 -> Gain9/1
  Gain9/1 -> Scope9/1, Mux/7
  Gain10/1 -> Scope10/1
  Derivative3/1 -> Gain10/1
  iL1/1 -> Derivative3/1, Unit Delay3/1, Gain5/1
  Gain11/1 -> Mux/9, Scope11/1
  L/1 -> Gain11/1

== matlab function DUs_Exp/Predict2 ==
  data: d1_hat input; d12_hat input; d13_hat input; d2_hat input; x1_star output; x2_star output; u_star output; V1cref input
function [x1_star,x2_star,u_star] = fcn(d1_hat,d12_hat,d13_hat,d2_hat, V1cref)
C = 0.0011;
L = 0.001;
R = 10000000;
E = 75;


%iL = (d1_hat+Vcref^2/R)/E;
 
x1_star = 0.5*C*V1cref^2+0.5*L*(d1_hat/E)^2;
x2_star =L/E^2*d1_hat*d12_hat-d1_hat;  
u_star = L/E^2*(d12_hat^2+d1_hat*d13_hat)-d12_hat-d2_hat;

== matlab function DUs_Exp/HOSM4 ==
  data: v input; z20 input; z21 input; z22 input; x2 input; z20_dot output; z21_dot output; lam2 input; z22_dot output

function [z20_dot,z21_dot,z22_dot] = fcn(v,z20,z21,z22,x2,lam2)

% l20 = 4;
% l21 = 2;
% l22=1;
l20 = 30;
l21 = 20;
l22 = 10;

h20 = -l20*lam2^(1/3)*abs(z20-x2)^(2/3)*sign(z20-x2)+z21; 
h21 = -l21*lam2^(1/2)*abs(z21-h20)^(1/2)*sign(z21-h20)+z22;     %h2,1
h22 = -l22*lam2*sign(z22-h21);                %h2,0
z20_dot = v+h20;                                 %z2,0的导数
z21_dot = h21;                                           %z2,1的导数 
z22_dot = h22;

== matlab function DUs_Exp/Predict1 ==
  data: d1_hat input; d12_hat input; d13_hat input; d2_hat input; x1_star output; x2_star output; u_star output; V2cref input
function [x1_star,x2_star,u_star] = fcn(d1_hat,d12_hat,d13_hat,d2_hat,V2cref)
C = 0.0011;
L = 0.001;
R = 10000000;
E = 75;
 

%iL = (d1_hat+Vcref^2/R)/E;
 
x1_star = 0.5*C*V2cref^2+0.5*L*(d1_hat/E)^2;
x2_star =L/E^2*d1_hat*d12_hat-d1_hat;  
u_star = L/E^2*(d12_hat^2+d1_hat*d13_hat)-d12_hat-d2_hat;

== matlab function DUs_Exp/controller2 ==
  data: v output; x1 input; x2 input; x1_star input; x2_star input; v_star input; k1 input; k2 input; tau input; L2 input
%计算虚拟控制律v
function v  = fcn(x1,x2,x1_star,x2_star,v_star,k1,k2,tau,L2)


q1 = x1-x1_star;
q2 = (x2-x2_star)/L2;

z = -k1*abs(q1)^(1+2*tau)*sign(q1)-k2*abs(q2)^((1+2*tau)/(1+tau))*sign(q2);

v = L2^2*z+v_star;

== matlab function DUs_Exp/duty4/MATLAB Function ==
  data: E input; mu output; L input; vc input; v input
function mu = fcn(E,L,vc,v)
mu=1-(E*E/L-v)/(vc*E/L);

== matlab function DUs_Exp/duty5/MATLAB Function ==
  data: E input; mu output; L input; vc input; v input
function mu = fcn(E,L,vc,v)
mu=1-(E*E/L-v)/(vc*E/L);

== matlab function DUs_Exp/HOSM1 ==
  data: lam1 input; z10 input; z11 input; z12 input; z13 input; x1 input; x2 input; z10_dot output; z11_dot output; z12_dot output; z13_dot output
%% 高阶滑模观测器1,l10,l11,l12,lam1为手动调的参数,返回z10,z11,z12的导数
function [z10_dot,z11_dot,z12_dot,z13_dot] = fcn(lam1,z10,z11,z12,z13,x1,x2)

% l0=5;
% l1=4;
% l2=2;
% l3=1;

% l0=60;
% l1=50;
% l2=40;
% l3=30;

l0=40;
l1=30;
l2=20;
l3=10;

h10=-l0*lam1^(1/4)*abs(z10-x1)^(3/4)*sign(z10-x1)+z11;
h11=-l1*lam1^(1/3)*abs(z11-h10)^(2/3)*sign(z11-h10)+z12;
h12=-l2*lam1^(1/2)*abs(z12-h11)^(1/2)*sign(z12-h11)+z13;
h13=-l3*lam1*sign(z13-h12);

z10_dot=x2+h10;
z11_dot=h11;
z12_dot=h12;
z13_dot=h13;

== matlab function DUs_Exp/controller3 ==
  data: v output; x1 input; x2 input; x1_star input; x2_star input; v_star input; k1 input; k2 input; tau input; L1 input
%计算虚拟控制律v
function v  = fcn(x1,x2,x1_star,x2_star,v_star,k1,k2,tau,L1)

q1 = x1-x1_star;
q2 = (x2-x2_star)/L1;

z = -k1*abs(q1)^(1+2*tau)*sign(q1)-k2*abs(q2)^((1+2*tau)/(1+tau))*sign(q2);

v = L1^2*z+v_star;

== matlab function DUs_Exp/HOSM3 ==
  data: lam1 input; z10 input; z11 input; z12 input; z13 input; x1 input; x2 input; z10_dot output; z11_dot output; z12_dot output; z13_dot output
%% 高阶滑模观测器1,l10,l11,l12,lam1为手动调的参数,返回z10,z11,z12的导数
function [z10_dot,z11_dot,z12_dot,z13_dot] = fcn(lam1,z10,z11,z12,z13,x1,x2)

% l0=60;
% l1=50;
% l2=40;
% l3=30;
l0=40;
l1=30;
l2=20;
l3=10;
% l0=5;
% l1=4;
% l2=2;
% l3=1;

h10=-l0*lam1^(1/4)*abs(z10-x1)^(3/4)*sign(z10-x1)+z11;
h11=-l1*lam1^(1/3)*abs(z11-h10)^(2/3)*sign(z11-h10)+z12;
h12=-l2*lam1^(1/2)*abs(z12-h11)^(1/2)*sign(z12-h11)+z13;
h13=-l3*lam1*sign(z13-h12);

z10_dot=x2+h10;
z11_dot=h11;
z12_dot=h12;
z13_dot=h13;

== matlab function DUs_Exp/HOSM2 ==
  data: v input; z20 input; z21 input; z22 input; x2 input; z20_dot output; z21_dot output; lam2 input; z22_dot output

function [z20_dot,z21_dot,z22_dot] = fcn(v,z20,z21,z22,x2,lam2)

l20 = 30;
l21 = 20;
l22=10;
% l20 = 4;
% l21 = 2;
% l22 = 1;

h20 = -l20*lam2^(1/3)*abs(z20-x2)^(2/3)*sign(z20-x2)+z21; 
h21 = -l21*lam2^(1/2)*abs(z21-h20)^(1/2)*sign(z21-h20)+z22;     %h2,1
h22 = -l22*lam2*sign(z22-h21);                %h2,0
z20_dot = v+h20;                                 %z2,0的导数
z21_dot = h21;                                           %z2,1的导数 
z22_dot = h22;
